simulink model "Planilla_3DOF_Crane"  (Simulink 7.8)
settings: Solver=FixedStepDiscrete  StartTime=0.0  StopTime=inf  FixedStep=0.01  RelTol=1e-3
values from neighbouring files (symbols this model uses):
  IMAX_AMP = 7    [setup.mat]
  K_CURR = -2    [setup.mat]
  K_ENC_ALPHA = 0.00153398078789    [setup.mat]
  K_ENC_GAMMA = 0.00153398078789    [setup.mat]
  K_ENC_THETA = 1.53398078789e-05    [setup.mat]
  K_ENC_X = -8.37996199324e-07    [setup.mat]
  K_ENC_Z = -6.95769857362e-07    [setup.mat]
  Ka = 0.5    [setup.mat]
  VMAX_DAC = 10    [setup.mat]
undefined symbols (not defined in the file or in its folder): HIL, jib_xref, qc_get_step_size, tower_xref
libraries: simulink x7, quarc_library x4, simulink_extras x3, mpclib x2
settings Model: Creator=MLevis  LastModifiedBy=UCH  SimulationMode=external  ExtModeTrigDuration=600000
settings SolverCC: PositivePriorityOrder=on  AutoInsertRateTranBlk=on
settings OptimizationCC: InitFltsAndDblsToZero=on
settings DebuggingCC: SaveWithParameterizedLinksMsg=none  FcnCallInpInsideContextMsg=Use local settings  StrictBusMsg=Warning
settings RTWCC: SystemTargetFile=quarc_win64.tlc  TemplateMakefile=quarc_default_tmf  Description=QUARC Win64 Target  ProcessScript=quarc_win64_make_rtw_hook
settings STFCustomTargetCC: TargetPreCompLibLocation=C:\PROGRA~3\QUARC\lib\2011b\win64\release  SystemTargetFile=quarc_win64.tlc
settings GRTTargetCC: TargetPreCompLibLocation=C:\PROGRA~3\QUARC\lib\2011b\win64\release  ParMdlRefBuildCompliant=off  CompOptLevelCompliant=off  ConcurrentExecutionCompliant=off  MatFileLogging=off  ExtMode=on  ExtModeMexFile=quarc_comm

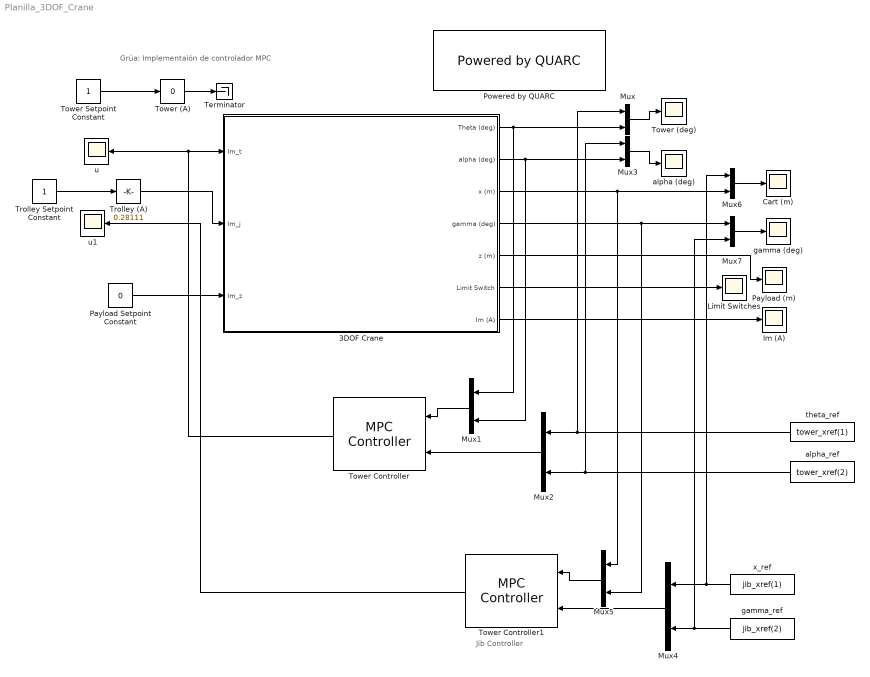
== system Planilla_3DOF_Crane ==
  note: Grúa: Implementaión de controlador MPC
  note: Jib Controller
  3DOF Crane : Subsystem
      mask Display:
      | image(imread('crane.png'))
      | port_label('input',1,'Im_t (A)','texmode','on')
      | port_label('input',2,'Im_j (A)','texmode','on')
      | port_label('input',3,'Im_z (A)','texmode','on')
      | 
      | port_label('output',1,'\theta (deg)','texmode','on')
      | port_label('output',2,'\alpha (deg)','texmode','on')
      | port_label('output',3,'x (m)','texmode','on')
      | port_label('output',4,'\gamma (deg)','texmode','on')
      | port_label('output',5,'z (m)','texmode','on')
      | port_label('output',6,'Limit Switches','texmode','on')
      | port_label('output',7,'Im (A)','texmode','on')
  Cart (m) : Scope
      settings: TimeRange=10  YMin=0.025  YMax=0.2  SaveName=x  DataFormat=Array
  Im (A) : Scope
      settings: YMin=-0.3  YMax=0.8  SaveName=Im  DataFormat=Array
  Limit Switches : Scope
      settings: YMin=-0.1  YMax=1.1  SaveName=Limit_Switches  DataFormat=Array
  Mux{,1..7} (8 alike) : Mux  Inputs=2
  Payload (m) : Scope
      settings: YMin=-0  YMax=0.2  SaveName=z  DataFormat=Array
  "Payload Setpoint Constant " : Constant  Value=0
  Powered by QUARC : quarc_library/Logos/Powered by QUARC
  Terminator : Terminator
  Tower (A) : simulink/Math Operations/Slider Gain  low=-0.5  gain=0  high=0.5
  Tower (deg) : Scope
      settings: YMin=60  YMax=180  SaveName=theta  DataFormat=Array
  Tower Controller : mpclib/MPC Controller  mpcobj=tower_MPC  x0=[]  ref_from_ws=off  ref_signal_name=[]  ref_preview=on  md_from_ws=off  md_signal_name=[]  md_preview=on  md_inport=off  mv_inport=off  lims_inport=off  switch_inport=off  ywt_inport=off  duwt_inport=off  rhoeps_inport=off  cost_outport=off  return_sequence=off  return_qpstatus=off  is_multiple=0  enable_value=0  n_mv=1  n_mo=2  n_md=0  n_ts=0.5  is_designfromscratch=0  from_project=off  project_file=MPCtask.mat
  Tower Controller1 : mpclib/MPC Controller  mpcobj=jib_MPC  x0=[]  ref_from_ws=off  ref_signal_name=[]  ref_preview=on  md_from_ws=off  md_signal_name=[]  md_preview=on  md_inport=off  mv_inport=off  lims_inport=off  switch_inport=off  ywt_inport=off  duwt_inport=off  rhoeps_inport=off  cost_outport=off  return_sequence=off  return_qpstatus=off  is_multiple=0  enable_value=0  n_mv=1  n_mo=2  n_md=0  n_ts=0.01  is_designfromscratch=0  from_project=off  project_file=MPCtask.mat
  "Tower Setpoint Constant " : Constant
  Trolley (A) : simulink/Math Operations/Slider Gain  low=-1  gain=0.28111  high=1
  "Trolley Setpoint Constant " : Constant
  alpha (deg) : Scope
      settings: YMin=0  YMax=32.5  SaveName=alpha  DataFormat=Array
  alpha_ref : Constant  Value=tower_xref(2)
  gamma (deg) : Scope
      settings: YMin=-25  YMax=25  SaveName=gamma  DataFormat=Array
  gamma_ref : Constant  Value=jib_xref(2)
  theta_ref : Constant  Value=tower_xref(1)
  u : Scope
      settings: YMin=1160.75  YMax=1282.93
  u1 : Scope
      settings: YMin=1160.75  YMax=1282.93
  x_ref : Constant  Value=jib_xref(1)
  wires:
  3DOF Crane/7(Im (A)) -> Im (A)/1
  3DOF Crane/5(z (m)) -> Payload (m)/1
  3DOF Crane/4(gamma (deg)) -> Mux5/2, Mux7/1
  3DOF Crane/3(x (m)) -> Mux5/1, Mux6/2
  3DOF Crane/2(alpha (deg)) -> Mux1/2, Mux3/2
  3DOF Crane/1(Theta (deg)) -> Mux1/1, Mux/2
  3DOF Crane/6(Limit Switch) -> Limit Switches/1
  Mux1/1 -> Tower Controller/1
  theta_ref/1 -> Mux2/1, Mux/1
  Mux2/1 -> Tower Controller/2
  alpha_ref/1 -> Mux2/2, Mux3/1
  Mux/1 -> Tower (deg)/1
  Mux3/1 -> alpha (deg)/1
  Tower Controller/1 -> u/1, 3DOF Crane/1(Im_t)
  "Tower Setpoint Constant "/1 -> Tower (A)/1
  Tower (A)/1 -> Terminator/1
  x_ref/1 -> Mux4/1, Mux6/1
  Mux4/1 -> Tower Controller1/2
  gamma_ref/1 -> Mux4/2, Mux7/2
  Mux5/1 -> Tower Controller1/1
  Mux6/1 -> Cart (m)/1
  Mux7/1 -> gamma (deg)/1
  "Trolley Setpoint Constant "/1 -> Trolley (A)/1
  Trolley (A)/1 -> 3DOF Crane/2(Im_j)
  Tower Controller1/1 -> u1/1
  "Payload Setpoint Constant "/1 -> 3DOF Crane/3(Im_z)

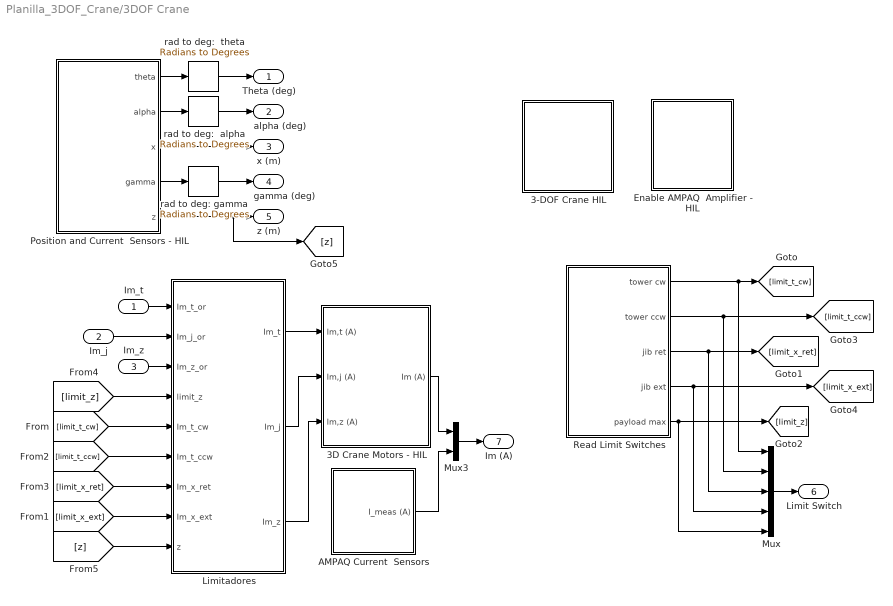
== system Planilla_3DOF_Crane/3DOF Crane ==
  Im_t : Inport
  Im_j : Inport  Port=2
  Im_z : Inport  Port=3
  3-DOF Crane HIL : Subsystem
  3D Crane Motors - HIL : Subsystem
  AMPAQ Current  Sensors : Subsystem
  Enable AMPAQ  Amplifier - HIL : Subsystem
  Limitadores : Subsystem
  Mux : Mux  Inputs=5
  Mux3 : Mux  Inputs=2
  Position and Current  Sensors - HIL : Subsystem
  Read Limit Switches : Subsystem
  rad to deg:  theta : simulink_extras/Transformations/Radians to Degrees
  rad to deg: gamma : simulink_extras/Transformations/Radians to Degrees
  rad to deg:  alpha : simulink_extras/Transformations/Radians to Degrees
  Theta (deg) : Outport
  alpha (deg) : Outport  Port=2
  x (m) : Outport  Port=3
  gamma (deg) : Outport  Port=4
  z (m) : Outport  Port=5
  Limit Switch : Outport  Port=6
  Im (A) : Outport  Port=7
  wires:
  rad to deg:  theta/1 -> Theta (deg)/1
  rad to deg:  alpha/1 -> alpha (deg)/1
  rad to deg: gamma/1 -> gamma (deg)/1
  Position and Current  Sensors - HIL/1(theta) -> rad to deg:  theta/1
  Position and Current  Sensors - HIL/2(alpha) -> rad to deg:  alpha/1
  Position and Current  Sensors - HIL/3(x) -> x (m)/1
  Position and Current  Sensors - HIL/4(gamma) -> rad to deg: gamma/1
  Position and Current  Sensors - HIL/5(z) -> z (m)/1, [z]
  Read Limit Switches/1(tower cw) -> Mux/1, [limit_t_cw]
  Read Limit Switches/3(jib ret) -> Mux/3, [limit_x_ret]
  Read Limit Switches/4(jib ext) -> Mux/4, [limit_x_ext]
  Read Limit Switches/2(tower ccw) -> Mux/2, [limit_t_ccw]
  AMPAQ Current  Sensors/1(I_meas (A)) -> Mux3/2
  3D Crane Motors - HIL/1(Im (A)) -> Mux3/1
  Mux3/1 -> Im (A)/1
  Mux/1 -> Limit Switch/1
  Read Limit Switches/5(payload max) -> Mux/5, [limit_z]
  Limitadores/3(Im_z) -> 3D Crane Motors - HIL/3(Im,z (A))
  Limitadores/1(Im_t) -> 3D Crane Motors - HIL/1(Im,t (A))
  Im_t/1 -> Limitadores/1(Im_t_or)
  [limit_z] -> Limitadores/4(limit_z)
  Im_z/1 -> Limitadores/3(Im_z_or)
  Im_j/1 -> Limitadores/2(Im_j_or)
  [limit_x_ret] -> Limitadores/7(Im_x_ret)
  [limit_x_ext] -> Limitadores/8(Im_x_ext)
  [limit_t_ccw] -> Limitadores/6(Im_t_ccw)
  [limit_t_cw] -> Limitadores/5(Im_t_cw)
  Limitadores/2(Im_j) -> 3D Crane Motors - HIL/2(Im,j (A))
  [z] -> Limitadores/9(z)

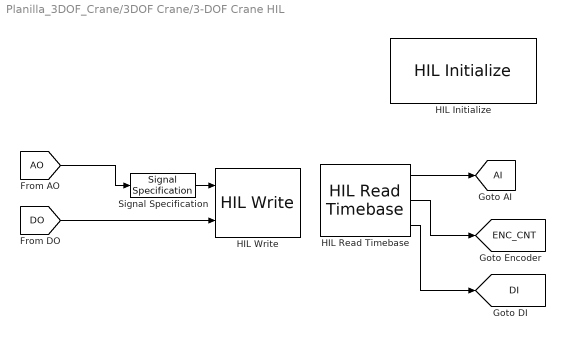
== system Planilla_3DOF_Crane/3DOF Crane/3-DOF Crane HIL ==
  HIL Initialize : quarc_library/Data Acquisition/Generic/Configuration/HIL Initialize  object_name=HIL-1  board_type=qpid  board_number=0  board_options=enc0_dir=0;enc0_filter=1;enc0_a=1;enc0_b=1;enc0_z=0;enc0_reload=0;enc1_dir=0;enc1_filter=1;enc1_a=1;enc1_b=1;enc1_z=0;enc1_reload=0;enc2_dir=0;enc2_filter=1;enc2_a=1;enc2_b=1;enc2_z=0;enc2_reload=0;enc3_dir=0;enc3_filter=1;enc3_a=1;enc3_b=1;enc3_z=0;enc3_reload=0;enc4_dir=0;enc4_filter=1;enc4_a=1;enc4_b=1;enc4_z=0;enc4_reload=0;enc5_dir=0;enc5_filter=1;enc5_a=1;enc5_b=1;enc5_z=0;enc5_reload=0;enc6_dir=0;enc6_filter=1;enc6_a=1;enc6_b=1;enc6_z=0;enc6_reload=0;enc7_dir=0;enc7_filter=1;enc7_a=1;enc7_b=1;enc7_z=0;enc7_reload=0;ext_int_polarity=0;fuse_polarity=0;convert_polarity=0;watchdog_polarity=0;ext_int_watchdog=0;fuse_watchdog=0;trig1_watchdog=0;watchdog_to_trig1=0;watchdog_to_trig2=0;counter_to_trig0=0;trigger_adcs=0;latch_on_adc=0;pwm_immediate=0  exclusive=off  active=on  hardware_clocks=[0:16]  clock_modes=[]  initial_clock_frequencies=[]  set_clock_params_at_start=off  set_clock_params_at_switch_in=off  set_clock_frequencies_at_start=off  set_clock_frequencies_at_switch_in=off  analog_input_channels=[0:7]  analog_input_maximums=10  analog_input_minimums=-10  set_analog_input_params_at_start=off  set_analog_input_params_at_switch_in=off  analog_output_channels=[0:7]  analog_output_maximums=10  analog_output_minimums=-10  initial_analog_outputs=[0]  final_analog_outputs=[0]  watchdog_analog_outputs=0  set_analog_output_params_at_start=off  set_analog_output_params_at_switch_in=off  set_analog_outputs_at_start=on  set_analog_outputs_at_switch_in=off  set_analog_outputs_at_terminate=on  set_analog_outputs_at_switch_out=off  set_analog_outputs_on_watchdog=off  digital_input_channels=[]  digital_output_channels=[]  digital_output_configuration=[]  initial_digital_outputs=[1]  final_digital_outputs=[1]  watchdog_digital_outputs=[2]  set_digital_output_params_at_start=off  set_digital_output_params_at_switch_in=off  set_digital_outputs_at_start=on  set_digital_outputs_at_switch_in=off  set_digital_outputs_at_terminate=on  set_digital_outputs_at_switch_out=off  set_digital_outputs_on_watchdog=off  encoder_channels=[0:7]  quadrature=[4]  encoder_filter_frequency=40e6/1  initial_encoder_counts=[0]  set_encoder_params_at_start=on  set_encoder_params_at_switch_in=off  set_encoder_counts_at_start=on  set_encoder_counts_at_switch_in=off  pwm_channels=[0:7]  pwm_modes=0  pwm_frequency=40e6/4096  pwm_configuration=[0]  pwm_alignment=[0]  pwm_polarity=[1]  pwm_leading_deadband=[0]  pwm_trailing_deadband=[0]  initial_pwm_outputs=[0]  final_pwm_outputs=[0]  watchdog_pwm_outputs=[0]  set_pwm_params_at_start=on  set_pwm_params_at_switch_in=off  set_pwm_outputs_at_start=on  set_pwm_outputs_at_switch_in=off  set_pwm_outputs_at_terminate=on  set_pwm_outputs_at_switch_out=off  set_pwm_outputs_on_watchdog=off  other_output_channels=[]  initial_other_outputs=[]  final_other_outputs=[]  watchdog_other_outputs=[]  set_other_outputs_at_start=off  set_other_outputs_at_switch_in=off  set_other_outputs_at_terminate=off  set_other_outputs_at_switch_out=off  set_other_outputs_on_watchdog=off
      settings: AttributesFormatString=%<object_name>
  HIL Read Timebase : quarc_library/Data Acquisition/Generic/Timebases/HIL Read Timebase  Tag=unassigned  object_name=HIL-1  clock=0  analog_channels=[0:2]  encoder_channels=[0:4]  digital_channels=[8:12]  other_channels=[]  samples_in_buffer=max(ceil(1/qc_get_step_size), 1)  active=on  vector_output=on  data_type_mode=Inherit via back propagation  encoder_data_type=double  digital_data_type=boolean
  HIL Write : quarc_library/Data Acquisition/Generic/Immediate I//O/HIL Write  Tag=unassigned  object_name=HIL-1  analog_channels=[0:2]  pwm_channels=[]  digital_channels=[0,1,2,4]  other_channels=[]  sample_time=-1  active=off  vector_input=on
  Signal Specification : SignalSpecification  OutDataTypeStr=double
  tag scope: AI=global, DI=global, ENC_CNT=global
  wires:
  HIL Read Timebase/3 -> [DI]
  HIL Read Timebase/1 -> [AI]
  HIL Read Timebase/2 -> [ENC_CNT]
  [DO] -> HIL Write/2
  [AO] -> Signal Specification/1
  Signal Specification/1 -> HIL Write/1

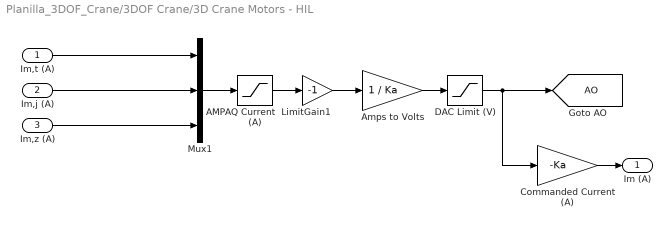
== system Planilla_3DOF_Crane/3DOF Crane/3D Crane Motors - HIL ==
  Im,t (A) : Inport
  Im,j (A) : Inport  Port=2
  Im,z (A) : Inport  Port=3
  AMPAQ Current  Limit (A) : Saturate  UpperLimit=IMAX_AMP  LowerLimit=-IMAX_AMP
  Amps to Volts : Gain  Gain=1 / Ka  SaturateOnIntegerOverflow=on  OutDataTypeStr=Inherit: Same as input  ParamDataTypeStr=Inherit: Same as input
  Commanded Current (A) : Gain  Gain=-Ka  SaturateOnIntegerOverflow=on  OutDataTypeStr=Inherit: Same as input  ParamDataTypeStr=Inherit: Same as input
  DAC Limit (V) : Saturate  UpperLimit=VMAX_DAC  LowerLimit=-VMAX_DAC
  Gain1 : Gain  Gain=-1
  Mux1 : Mux  Inputs=3
  Im (A) : Outport
  tag scope: AO=global
  wires:
  Im,z (A)/1 -> Mux1/3
  Im,t (A)/1 -> Mux1/1
  AMPAQ Current  Limit (A)/1 -> Gain1/1
  Mux1/1 -> AMPAQ Current  Limit (A)/1
  DAC Limit (V)/1 -> [AO], Commanded Current (A)/1
  Amps to Volts/1 -> DAC Limit (V)/1
  Im,j (A)/1 -> Mux1/2
  Gain1/1 -> Amps to Volts/1
  Commanded Current (A)/1 -> Im (A)/1

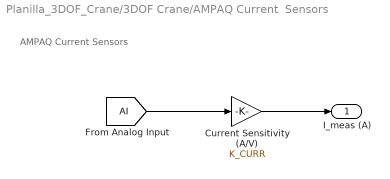
== system Planilla_3DOF_Crane/3DOF Crane/AMPAQ Current  Sensors ==
  note: AMPAQ Current Sensors
  Current Sensitivity (A/V) : Gain  Gain=K_CURR
  I_meas (A) : Outport
  wires:
  Current Sensitivity (A/V)/1 -> I_meas (A)/1
  [AI] -> Current Sensitivity (A/V)/1

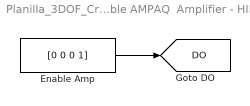
== system Planilla_3DOF_Crane/3DOF Crane/Enable AMPAQ  Amplifier - HIL ==
  Enable Amp : Constant  Value=[0 0 0 1]
  tag scope: DO=global
  wires:
  Enable Amp/1 -> [DO]

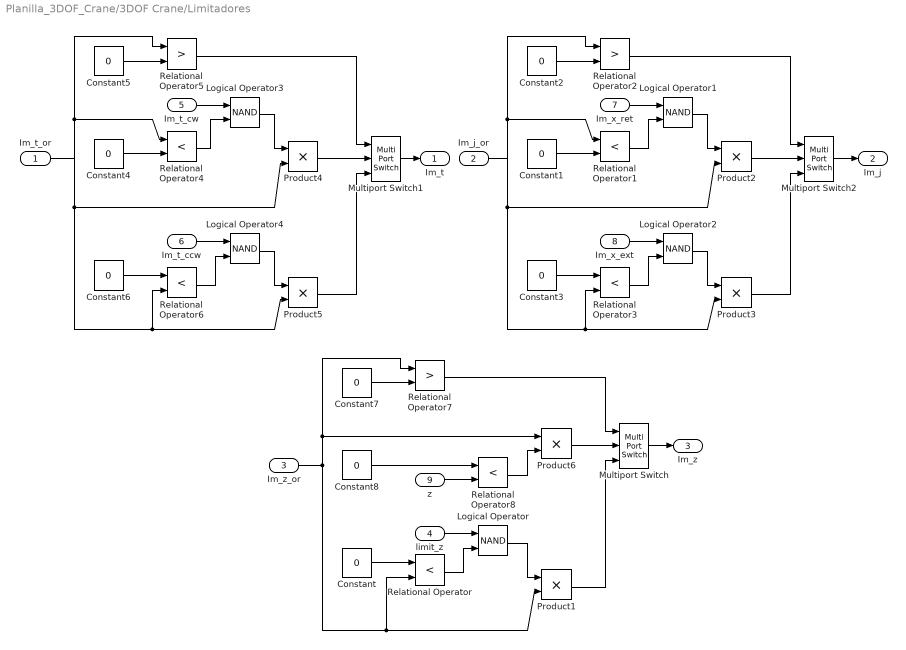
== system Planilla_3DOF_Crane/3DOF Crane/Limitadores ==
  Im_t_or : Inport
  Im_j_or : Inport  Port=2
  Im_z_or : Inport  Port=3
  limit_z : Inport  Port=4
  Im_t_cw : Inport  Port=5
  Im_t_ccw : Inport  Port=6
  Im_x_ret : Inport  Port=7
  Im_x_ext : Inport  Port=8
  z : Inport  Port=9
  Constant{,1..8} (9 alike) : Constant  Value=0
  Logical Operator{,1..4} (5 alike) : Logic  Operator=NAND  AllPortsSameDT=off  OutDataTypeStr=boolean
  Multiport Switch : MultiPortSwitch  DataPortOrder=Zero-based contiguous  Inputs=2  zeroidx=on
  Multiport Switch1 : MultiPortSwitch  DataPortOrder=Zero-based contiguous  Inputs=2  zeroidx=on
  Multiport Switch2 : MultiPortSwitch  DataPortOrder=Zero-based contiguous  Inputs=2  zeroidx=on
  Product{1..6} (6 alike) : Product  RndMeth=Zero
  Relational Operator{,1,3..4,6,8} (6 alike) : RelationalOperator  Operator=<  OutDataTypeStr=boolean
  Relational Operator2 : RelationalOperator  Operator=>  OutDataTypeStr=boolean
  Relational Operator5 : RelationalOperator  Operator=>  OutDataTypeStr=boolean
  Relational Operator7 : RelationalOperator  Operator=>  OutDataTypeStr=boolean
  Im_t : Outport
  Im_j : Outport  Port=2
  Im_z : Outport  Port=3
  wires:
  Constant/1 -> Relational Operator/1
  limit_z/1 -> Logical Operator/1
  Relational Operator/1 -> Logical Operator/2
  Logical Operator/1 -> Product1/1
  Product1/1 -> Multiport Switch/3
  Im_j_or/1 -> Relational Operator1/1, Product2/2, Relational Operator3/2, Product3/2, Relational Operator2/1
  Constant2/1 -> Relational Operator2/2
  Relational Operator2/1 -> Multiport Switch2/1
  Constant3/1 -> Relational Operator3/1
  Im_x_ext/1 -> Logical Operator2/1
  Relational Operator3/1 -> Logical Operator2/2
  Logical Operator2/1 -> Product3/1
  Product3/1 -> Multiport Switch2/3
  Im_x_ret/1 -> Logical Operator1/1
  Relational Operator1/1 -> Logical Operator1/2
  Logical Operator1/1 -> Product2/1
  Constant1/1 -> Relational Operator1/2
  Product2/1 -> Multiport Switch2/2
  Multiport Switch2/1 -> Im_j/1
  Im_t_or/1 -> Relational Operator4/1, Product4/2, Relational Operator6/2, Product5/2, Relational Operator5/1
  Constant5/1 -> Relational Operator5/2
  Relational Operator5/1 -> Multiport Switch1/1
  Constant6/1 -> Relational Operator6/1
  Im_t_ccw/1 -> Logical Operator4/1
  Relational Operator6/1 -> Logical Operator4/2
  Logical Operator4/1 -> Product5/1
  Product5/1 -> Multiport Switch1/3
  Im_t_cw/1 -> Logical Operator3/1
  Relational Operator4/1 -> Logical Operator3/2
  Logical Operator3/1 -> Product4/1
  Constant4/1 -> Relational Operator4/2
  Product4/1 -> Multiport Switch1/2
  Multiport Switch1/1 -> Im_t/1
  Im_z_or/1 -> Relational Operator/2, Product1/2, Relational Operator7/1, Product6/1
  Constant7/1 -> Relational Operator7/2
  Relational Operator7/1 -> Multiport Switch/1
  Multiport Switch/1 -> Im_z/1
  Constant8/1 -> Relational Operator8/1
  z/1 -> Relational Operator8/2
  Relational Operator8/1 -> Product6/2
  Product6/1 -> Multiport Switch/2

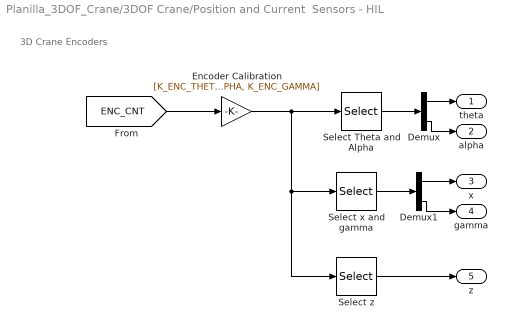
== system Planilla_3DOF_Crane/3DOF Crane/Position and Current  Sensors - HIL ==
  note: 3D Crane Encoders
  Demux : Demux  Outputs=2
  Demux1 : Demux  Outputs=2
  Encoder Calibration : Gain  Gain=[K_ENC_THETA, K_ENC_X, K_ENC_Z, K_ENC_ALPHA, K_ENC_GAMMA]
  Select Theta and Alpha : Selector  InputPortWidth=5  IndexOptions=Index vector (dialog)  Indices=[1, 4]  OutputSizes=1
  Select x and gamma : Selector  InputPortWidth=5  IndexOptions=Index vector (dialog)  Indices=[2, 5]  OutputSizes=1
  Select z : Selector  InputPortWidth=5  IndexOptions=Index vector (dialog)  Indices=3  OutputSizes=1
  theta : Outport
  alpha : Outport  Port=2
  x : Outport  Port=3
  gamma : Outport  Port=4
  z : Outport  Port=5
  wires:
  [ENC_CNT] -> Encoder Calibration/1
  Select Theta and Alpha/1 -> Demux/1
  Select x and gamma/1 -> Demux1/1
  Demux/1 -> theta/1
  Demux/2 -> alpha/1
  Demux1/1 -> x/1
  Demux1/2 -> gamma/1
  Select z/1 -> z/1
  Encoder Calibration/1 -> Select Theta and Alpha/1, Select x and gamma/1, Select z/1

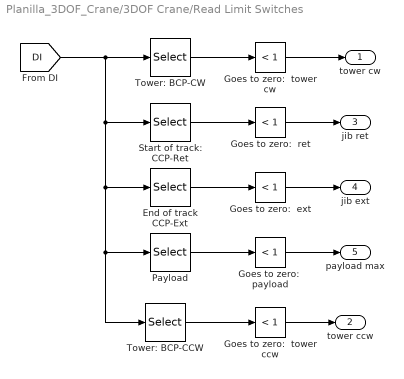
== system Planilla_3DOF_Crane/3DOF Crane/Read Limit Switches ==
  End of track CCP-Ext : Selector  InputPortWidth=5  IndexOptions=Index vector (dialog)  Indices=3  OutputSizes=1
  Goes to zero:  ext : simulink/Logic and Bit Operations/Compare To Constant  relop=<  const=1  OutDataTypeStr=boolean  ZeroCross=off
  Goes to zero:  payload : simulink/Logic and Bit Operations/Compare To Constant  relop=<  const=1  OutDataTypeStr=boolean  ZeroCross=off
  Goes to zero:  ret : simulink/Logic and Bit Operations/Compare To Constant  relop=<  const=1  OutDataTypeStr=boolean  ZeroCross=off
  Goes to zero:  tower ccw : simulink/Logic and Bit Operations/Compare To Constant  relop=<  const=1  OutDataTypeStr=boolean  ZeroCross=off
  Goes to zero:  tower cw : simulink/Logic and Bit Operations/Compare To Constant  relop=<  const=1  OutDataTypeStr=boolean  ZeroCross=off
  Payload : Selector  InputPortWidth=5  IndexOptions=Index vector (dialog)  Indices=4  OutputSizes=1
  Start of track: CCP-Ret : Selector  InputPortWidth=5  IndexOptions=Index vector (dialog)  Indices=2  OutputSizes=1
  Tower: BCP-CCW : Selector  InputPortWidth=5  IndexOptions=Index vector (dialog)  Indices=5  OutputSizes=1
  Tower: BCP-CW : Selector  InputPortWidth=5  IndexOptions=Index vector (dialog)  Indices=1  OutputSizes=1
  tower cw : Outport
  tower ccw : Outport  Port=2
  jib ret : Outport  Port=3
  jib ext : Outport  Port=4
  payload max : Outport  Port=5
  wires:
  [DI] -> End of track CCP-Ext/1, Payload/1, Tower: BCP-CCW/1, Start of track: CCP-Ret/1, Tower: BCP-CW/1
  Payload/1 -> Goes to zero:  payload/1
  Goes to zero:  payload/1 -> payload max/1
  Goes to zero:  tower cw/1 -> tower cw/1
  Tower: BCP-CW/1 -> Goes to zero:  tower cw/1
  Goes to zero:  ret/1 -> jib ret/1
  Goes to zero:  ext/1 -> jib ext/1
  Start of track: CCP-Ret/1 -> Goes to zero:  ret/1
  End of track CCP-Ext/1 -> Goes to zero:  ext/1
  Tower: BCP-CCW/1 -> Goes to zero:  tower ccw/1
  Goes to zero:  tower ccw/1 -> tower ccw/1
